simulink model "MBD_W1_P3"  (R2020a)
settings: Solver=VariableStepAuto  StartTime=0.0  StopTime=10.0  MaxStep=0.00001  RelTol=1e-3
settings Model: Creator=Atri Mondal  LastModifiedBy=Atri Mondal

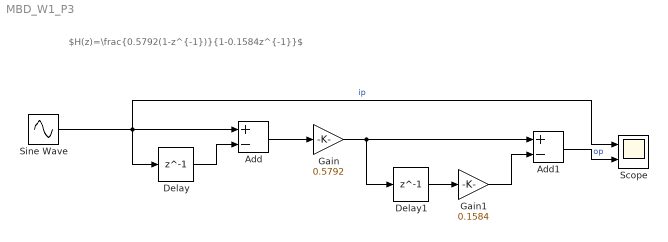
== system MBD_W1_P3 ==
  note: $H(z)=\frac{0.5792(1-z^{-1})}{1-0.1584z^{-1}}$
  Add : Sum  Inputs=+-
  Add1 : Sum  Inputs=+-
  Delay : Delay  DelayLength=1
  Delay1 : Delay  DelayLength=1
  Gain : Gain  Gain=0.5792
  Gain1 : Gain  Gain=0.1584
  Scope : Scope  NumInputPorts=2
  Sine Wave : Sin  Frequency=2*pi*1000  SampleTime=0
  wires:
  Sine Wave/1 -> Scope/1, Delay/1, Add/1  "ip"
  Delay/1 -> Add/2
  Add/1 -> Gain/1
  Gain/1 -> Delay1/1, Add1/1
  Delay1/1 -> Gain1/1
  Gain1/1 -> Add1/2
  Add1/1 -> Scope/2  "op"
